simulink model "tr_trim_VTAOAS"  (R2025a)
settings: Solver=VariableStepAuto  StartTime=0.0  StopTime=10.0  RelTol=1e-3
values from neighbouring files (symbols this model uses):
  const = load_const    [vtol_trim_lin_analysis.m]
  q = X(8)    [fixedwing_6dof_dynamics.m]    (also in fixedwing_trim_dynamics.m; fw_linearization_dynamics.m; fw_trim_dynamics.m; tr_linearization_dynamics.m)
  r = X(9)    [fixedwing_6dof_dynamics.m]    (also in fixedwing_trim_dynamics.m; fw_linearization_dynamics.m; fw_trim_dynamics.m; tr_linearization_dynamics.m)
  uavParam = load_vtol_dynamics_7000lb    [vtol_trim_lin_analysis.m]
undefined symbols (not defined in the file or in its folder): contact, env, F, flap_trim, H_trim, Light, MIL, tiltIni, uavParams
libraries: matrix_library x8, robotcorelib x4, aerolibasang x2, aerolibwind2 x2, aerolibadyn x1, sharedutil x1, aerolibatmos2 x1, sharedtransform x1
(part 2 of 2)

== system tr_trim_VTAOAS/Force and Moments/Aerodynamic Forces/Compute Body Frame Forces and Moments/Wind frame F& M/Lateral Channel/Cl ==
  alpha : Inport
  beta : Inport  Port=2
  dA : Inport  Port=3
  dR : Inport  Port=4
  p,q,r : Inport  Port=5
  Airspeed : Inport  Port=6
  1-D Lookup Table : Lookup_n-D  BreakpointsForDimension1=uavParams.aero.beta_latdir  BreakpointsForDimension2=uavParams.aero.alpha_latdir  Table=uavParams.aero.CR  InternalRulePriority=Speed  RndMeth=Simplest
      settings: InputPortMap=u0,u1
  Abs : Abs  Commented=on  SaturateOnIntegerOverflow=off
  ClDa : Constant  Value=uavParams.aero.ClDa
      settings: AttributesFormatString=%<Value>
  ClDr : Constant  Value=uavParams.aero.ClDr
      settings: AttributesFormatString=%<Value>
  Clb : Constant  Commented=on  Value=uavParam.aero.Clb
      settings: AttributesFormatString=%<Value>
  Product1 : Product  SaturateOnIntegerOverflow=on  OutDataTypeStr=Inherit: Same as first input
  Product2 : Product  Commented=on
  Product5 : Product  SaturateOnIntegerOverflow=on  OutDataTypeStr=Inherit: Same as first input
  Sign : Signum  Commented=on
  Sum : Sum  Inputs=+++++  SaturateOnIntegerOverflow=on
  roll factors : Subsystem
  Cl : Outport  VectorParamsAs1DForOutWhenUnconnected=off
  wires:
  roll factors/1(Clp) -> Sum/4
  Product5/1 -> Sum/2  "CldA"
  Airspeed/1 -> roll factors/2(Airspeed)
  p,q,r/1 -> roll factors/1(p,q,r)
  roll factors/2(Clr) -> Sum/5
  Product1/1 -> Sum/3  "Cldr"
  Sum/1 -> Cl/1
  dR/1 -> Product1/2
  ClDr/1 -> Product1/1
  dA/1 -> Product5/2
  ClDa/1 -> Product5/1
  Clb/1 -> ?
  Sign/1 -> Product2/2
  1-D Lookup Table/1 -> Sum/1  "Clb"
  beta/1 -> 1-D Lookup Table/1
  alpha/1 -> 1-D Lookup Table/2

== system tr_trim_VTAOAS/Force and Moments/Aerodynamic Forces/Compute Body Frame Forces and Moments/Wind frame F& M/Lateral Channel/Cn ==
  alpha : Inport
  beta : Inport  Port=2
  dA : Inport  Port=3
  dR : Inport  Port=4
  p,q,r : Inport  Port=5
  Airspeed : Inport  Port=6
  1-D Lookup Table : Lookup_n-D  BreakpointsForDimension1=uavParams.aero.beta_latdir  BreakpointsForDimension2=uavParams.aero.alpha_latdir  Table=uavParams.aero.CN  ExtrapMethod=Clip  UseLastTableValue=on  InternalRulePriority=Speed  RndMeth=Simplest
      settings: InputPortMap=u0,u1
  Abs : Abs  Commented=on  SaturateOnIntegerOverflow=off
  CnDa : Constant  Value=uavParams.aero.CnDa
      settings: AttributesFormatString=%<Value>
  CnDr : Constant  Value=uavParams.aero.CnDr
      settings: AttributesFormatString=%<Value>
  Cnb : Constant  Commented=on  Value=uavParam.aero.Cnb
      settings: AttributesFormatString=%<Value>
  Product1 : Product  SaturateOnIntegerOverflow=on  OutDataTypeStr=Inherit: Same as first input
  Product2 : Product  Commented=on
  Product5 : Product  SaturateOnIntegerOverflow=on  OutDataTypeStr=Inherit: Same as first input
  Sign : Signum  Commented=on
  Sum : Sum  Inputs=+++++  SaturateOnIntegerOverflow=on
  yaw factors : Subsystem
  Cn : Outport  VectorParamsAs1DForOutWhenUnconnected=off
  wires:
  Airspeed/1 -> yaw factors/2(Airspeed)
  p,q,r/1 -> yaw factors/1(p,q,r)
  CnDa/1 -> Product5/1
  Product5/1 -> Sum/2
  dA/1 -> Product5/2
  CnDr/1 -> Product1/1
  dR/1 -> Product1/2
  Sum/1 -> Cn/1
  Product1/1 -> Sum/3
  yaw factors/2(Cnr) -> Sum/5
  yaw factors/1(Cnp) -> Sum/4
  1-D Lookup Table/1 -> Sum/1
  Sign/1 -> Product2/2
  alpha/1 -> 1-D Lookup Table/2
  beta/1 -> 1-D Lookup Table/1

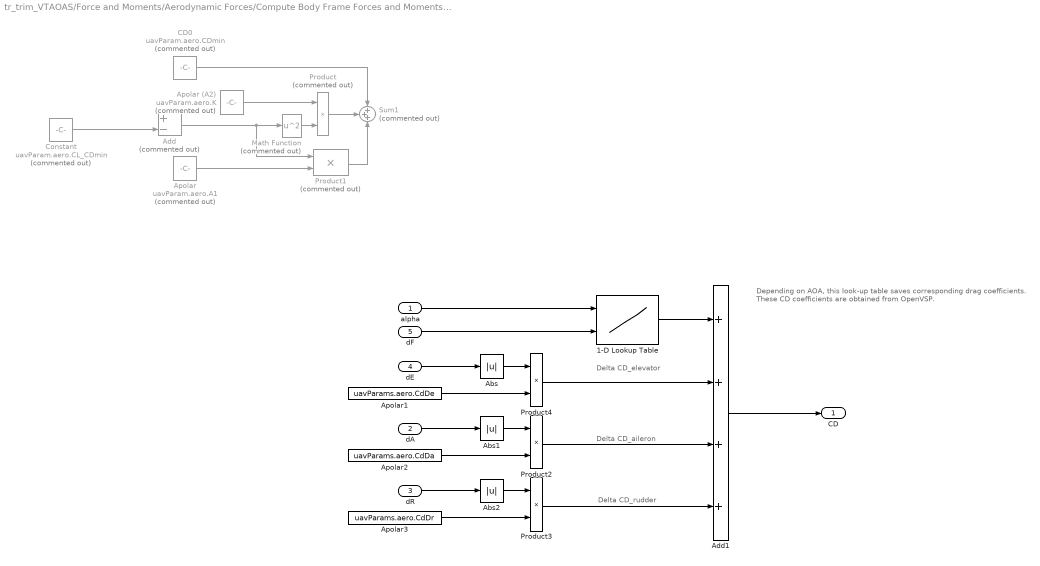
== system tr_trim_VTAOAS/Force and Moments/Aerodynamic Forces/Compute Body Frame Forces and Moments/Wind frame F& M/Longitudinal Channel/CD ==
  note: Delta CD_elevator
  note: Depending on AOA, this look-up table saves corresponding drag coefficients.
      | These CD coefficients are obtained from OpenVSP.
  note: Delta CD_aileron
  note: Delta CD_rudder
  alpha : Inport
  dA : Inport  Port=2
  dR : Inport  Port=3
  dE : Inport  Port=4
  dF : Inport  Port=5
  1-D Lookup Table : Lookup_n-D  BreakpointsForDimension1=uavParams.aero.alpha_lon  BreakpointsForDimension2=uavParams.aero.flap_lon  Table=uavParams.aero.CD  ExtrapMethod=Clip  UseLastTableValue=on  InternalRulePriority=Speed  RndMeth=Simplest
      settings: InputPortMap=u0,u1
  Abs : Abs  SaturateOnIntegerOverflow=off
  Abs1 : Abs  SaturateOnIntegerOverflow=off
  Abs2 : Abs  SaturateOnIntegerOverflow=off
  Add : Sum  Commented=on  Inputs=+-
  Add1 : Sum  Inputs=++++
  Apolar : Constant  Commented=on  Value=uavParam.aero.A1
      settings: AttributesFormatString=%<Value>
  Apolar (A2) : Constant  Commented=on  Value=uavParam.aero.K
      settings: AttributesFormatString=%<Value>
  Apolar1 : Constant  Value=uavParams.aero.CdDe
      settings: AttributesFormatString=%<Value>
  Apolar2 : Constant  Value=uavParams.aero.CdDa
      settings: AttributesFormatString=%<Value>
  Apolar3 : Constant  Value=uavParams.aero.CdDr
      settings: AttributesFormatString=%<Value>
  CD0 : Constant  Commented=on  Value=uavParam.aero.CDmin
      settings: AttributesFormatString=%<Value>
  Constant : Constant  Commented=on  Value=uavParam.aero.CL_CDmin
  Math Function : Math  Commented=on  Operator=square  SignedPower=on
  Product : Product  Commented=on  SaturateOnIntegerOverflow=on  OutDataTypeStr=Inherit: Same as first input
  Product1 : Product  Commented=on  SaturateOnIntegerOverflow=on  OutDataTypeStr=Inherit: Same as first input
  Product2 : Product  SaturateOnIntegerOverflow=on  OutDataTypeStr=Inherit: Same as first input
  Product3 : Product  SaturateOnIntegerOverflow=on  OutDataTypeStr=Inherit: Same as first input
  Product4 : Product  SaturateOnIntegerOverflow=on  OutDataTypeStr=Inherit: Same as first input
  Sum1 : Sum  Commented=on  Inputs=+++  SaturateOnIntegerOverflow=on
  CD : Outport  VectorParamsAs1DForOutWhenUnconnected=off
  wires:
  Add1/1 -> CD/1
  Apolar (A2)/1 -> Product/1
  Math Function/1 -> Product/2
  Product1/1 -> Sum1/3
  Product/1 -> Sum1/2
  Add/1 -> Product1/1, Math Function/1
  CD0/1 -> Sum1/1
  Apolar/1 -> Product1/2
  Constant/1 -> Add/2
  Apolar1/1 -> Product4/2
  dE/1 -> Abs/1
  Abs/1 -> Product4/1
  Abs1/1 -> Product2/1
  Apolar2/1 -> Product2/2
  dA/1 -> Abs1/1
  Abs2/1 -> Product3/1
  Apolar3/1 -> Product3/2
  dR/1 -> Abs2/1
  Product4/1 -> Add1/2
  Product2/1 -> Add1/3
  Product3/1 -> Add1/4
  1-D Lookup Table/1 -> Add1/1
  dF/1 -> 1-D Lookup Table/2
  alpha/1 -> 1-D Lookup Table/1

== system tr_trim_VTAOAS/Force and Moments/Aerodynamic Forces/Compute Body Frame Forces and Moments/Wind frame F& M/Longitudinal Channel/CL ==
  alpha : Inport
  alpha_dot : Inport  Port=2
  dE : Inport  Port=3
  p,q,r : Inport  Port=4
  Airspeed : Inport  Port=5
  dA : Inport  Port=6
  dF : Inport  Port=7
  1-D Lookup Table : Lookup_n-D  BreakpointsForDimension1=uavParams.aero.alpha_lon  BreakpointsForDimension2=uavParams.aero.flap_lon  Table=uavParams.aero.CL  ExtrapMethod=Clip  UseLastTableValue=on  InternalRulePriority=Speed  RndMeth=Simplest
      settings: InputPortMap=u0,u1
  Abs : Abs  SaturateOnIntegerOverflow=off
  CL1 : Constant  Value=uavParams.aero.CLDa
      settings: AttributesFormatString=%<Value>
  CLDe : Constant  Value=uavParams.aero.CLDe
      settings: AttributesFormatString=%<Value>
  CLa_dot : Constant  Value=uavParams.aero.CLadot
      settings: AttributesFormatString=%<Value>
  Lift due to pitch rate : Subsystem
  Product1 : Product  SaturateOnIntegerOverflow=on  OutDataTypeStr=Inherit: Same as first input
  Product2 : Product  SaturateOnIntegerOverflow=on  OutDataTypeStr=Inherit: Same as first input
  Product5 : Product  SaturateOnIntegerOverflow=on  OutDataTypeStr=Inherit: Same as first input
  Sum : Sum  Inputs=+++++  SaturateOnIntegerOverflow=on
  CL : Outport  VectorParamsAs1DForOutWhenUnconnected=off
  wires:
  Airspeed/1 -> Lift due to pitch rate/2(Airspeed)
  p,q,r/1 -> Lift due to pitch rate/1(p,q,r)
  Sum/1 -> CL/1
  dE/1 -> Product1/2
  CLDe/1 -> Product1/1
  alpha_dot/1 -> Product5/2
  CLa_dot/1 -> Product5/1
  CL1/1 -> Product2/2
  dA/1 -> Abs/1
  Abs/1 -> Product2/1
  Product5/1 -> Sum/2
  Lift due to pitch rate/1(CLq) -> Sum/5
  Product1/1 -> Sum/3
  Product2/1 -> Sum/4
  1-D Lookup Table/1 -> Sum/1
  alpha/1 -> 1-D Lookup Table/1
  dF/1 -> 1-D Lookup Table/2

== system tr_trim_VTAOAS/Force and Moments/Aerodynamic Forces/Compute Body Frame Forces and Moments/Wind frame F& M/Longitudinal Channel/Cm ==
  alpha : Inport
  dE : Inport  Port=2
  p,q,r : Inport  Port=3
  Airspeed : Inport  Port=4
  dF : Inport  Port=5
  1-D Lookup Table : Lookup_n-D  BreakpointsForDimension1=uavParams.aero.alpha_lon  BreakpointsForDimension2=uavParams.aero.flap_lon  Table=uavParams.aero.CM  ExtrapMethod=Clip  UseLastTableValue=on  InternalRulePriority=Speed  RndMeth=Simplest
      settings: InputPortMap=u0,u1
  CmDe : Constant  Value=uavParams.aero.CmDe
      settings: AttributesFormatString=%<Value>
  Lift due to pitch rate : Subsystem
  Product1 : Product  Inputs=**  SaturateOnIntegerOverflow=on  OutDataTypeStr=Inherit: Same as first input
  Sum : Sum  Inputs=+++  SaturateOnIntegerOverflow=on
  Cm : Outport  VectorParamsAs1DForOutWhenUnconnected=off
  wires:
  Lift due to pitch rate/1(Cmq) -> Sum/3  "cmq"
  p,q,r/1 -> Lift due to pitch rate/1(p,q,r)
  Sum/1 -> Cm/1  "total"
  dE/1 -> Product1/2
  CmDe/1 -> Product1/1
  Airspeed/1 -> Lift due to pitch rate/2(Airspeed)
  Product1/1 -> Sum/2  "cmde"
  alpha/1 -> 1-D Lookup Table/1
  1-D Lookup Table/1 -> Sum/1  "cma"
  dF/1 -> 1-D Lookup Table/2

== system tr_trim_VTAOAS/Force and Moments/Aerodynamic Forces/Compute Body Frame Forces and Moments/Wind frame F& M/Lateral Channel/CY/roll factors ==
  p,q,r : Inport
  Airspeed : Inport  Port=2
  Constant : Constant  Value=uavParams.aero.CYp
      settings: AttributesFormatString=%<Value>
  Constant1 : Constant  Value=uavParams.aero.CYr
      settings: AttributesFormatString=%<Value>
  Product : Product  SaturateOnIntegerOverflow=on  OutDataTypeStr=Inherit: Same as first input
  Product1 : Product  SaturateOnIntegerOverflow=on  OutDataTypeStr=Inherit: Same as first input
  Selector : Selector  InputPortWidth=3  IndexOptions=Index vector (dialog)  Indices=[1]  OutputSizes=1
  Selector1 : Selector  InputPortWidth=3  IndexOptions=Index vector (dialog)  Indices=[3]  OutputSizes=1
  Subsystem : Subsystem
  roll rate fact : Subsystem
  CSp : Outport  VectorParamsAs1DForOutWhenUnconnected=off
  CSr : Outport  Port=2  VectorParamsAs1DForOutWhenUnconnected=off
  wires:
  Selector1/1 -> Subsystem/1(r)
  p,q,r/1 -> Selector1/1, Selector/1
  Selector/1 -> roll rate fact/1(p)
  Airspeed/1 -> Subsystem/2(Airspeed), roll rate fact/2(Airspeed)
  Subsystem/1(Yaw Rate Fac) -> Product1/2
  roll rate fact/1(Roll Rate Fac) -> Product/2
  Product1/1 -> CSr/1
  Product/1 -> CSp/1
  Constant/1 -> Product/1
  Constant1/1 -> Product1/1

== system tr_trim_VTAOAS/Force and Moments/Aerodynamic Forces/Compute Body Frame Forces and Moments/Wind frame F& M/Lateral Channel/Cl/roll factors ==
  p,q,r : Inport
  Airspeed : Inport  Port=2
  Constant : Constant  Value=uavParams.aero.Clp
      settings: AttributesFormatString=%<Value>
  Constant1 : Constant  Value=uavParams.aero.Clr
      settings: AttributesFormatString=%<Value>
  Product : Product  SaturateOnIntegerOverflow=on  OutDataTypeStr=Inherit: Same as first input
  Product1 : Product  SaturateOnIntegerOverflow=on  OutDataTypeStr=Inherit: Same as first input
  Selector : Selector  InputPortWidth=3  IndexOptions=Index vector (dialog)  Indices=[1]  OutputSizes=1
  Selector1 : Selector  InputPortWidth=3  IndexOptions=Index vector (dialog)  Indices=[3]  OutputSizes=1
  roll rate fact : Subsystem
  yaw rate fact : Subsystem
  Clp : Outport  VectorParamsAs1DForOutWhenUnconnected=off
  Clr : Outport  Port=2  VectorParamsAs1DForOutWhenUnconnected=off
  wires:
  Selector1/1 -> yaw rate fact/1(r)
  p,q,r/1 -> Selector1/1, Selector/1
  Selector/1 -> roll rate fact/1(p)
  Airspeed/1 -> roll rate fact/2(Airspeed), yaw rate fact/2(Airspeed)
  yaw rate fact/1(Yaw Rate Fac) -> Product1/2
  Constant1/1 -> Product1/1
  roll rate fact/1(Roll Rate Fac) -> Product/2
  Constant/1 -> Product/1
  Product1/1 -> Clr/1
  Product/1 -> Clp/1

== system tr_trim_VTAOAS/Force and Moments/Aerodynamic Forces/Compute Body Frame Forces and Moments/Wind frame F& M/Lateral Channel/Cn/yaw factors ==
  p,q,r : Inport
  Airspeed : Inport  Port=2
  Constant : Constant  Value=uavParams.aero.Cnp
      settings: AttributesFormatString=%<Value>
  Constant1 : Constant  Value=uavParams.aero.Cnr
      settings: AttributesFormatString=%<Value>
  Product : Product  SaturateOnIntegerOverflow=on  OutDataTypeStr=Inherit: Same as first input
  Product1 : Product  SaturateOnIntegerOverflow=on  OutDataTypeStr=Inherit: Same as first input
  Selector : Selector  InputPortWidth=3  IndexOptions=Index vector (dialog)  Indices=[3]  OutputSizes=1
  Selector1 : Selector  InputPortWidth=3  IndexOptions=Index vector (dialog)  Indices=[1]  OutputSizes=1
  roll rate fact : Subsystem
  yaw rate fact1 : Subsystem
  Cnp : Outport  VectorParamsAs1DForOutWhenUnconnected=off
  Cnr : Outport  Port=2  VectorParamsAs1DForOutWhenUnconnected=off
  wires:
  Airspeed/1 -> yaw rate fact1/2(Airspeed), roll rate fact/2(Airspeed)
  Selector/1 -> yaw rate fact1/1(r)
  p,q,r/1 -> Selector1/1, Selector/1
  Selector1/1 -> roll rate fact/1(p)
  roll rate fact/1(Roll Rate Fac) -> Product/2
  Constant/1 -> Product/1
  yaw rate fact1/1(Yaw Rate Fac) -> Product1/2
  Constant1/1 -> Product1/1
  Product1/1 -> Cnr/1
  Product/1 -> Cnp/1

== system tr_trim_VTAOAS/Force and Moments/Aerodynamic Forces/Compute Body Frame Forces and Moments/Wind frame F& M/Longitudinal Channel/CL/Lift due to pitch rate ==
  p,q,r : Inport
  Airspeed : Inport  Port=2
  Constant : Constant  Value=uavParams.aero.CLq
      settings: AttributesFormatString=%<Value>
  Product : Product  SaturateOnIntegerOverflow=on  OutDataTypeStr=Inherit: Same as first input
  Selector : Selector  InputPortWidth=3  IndexOptions=Index vector (dialog)  Indices=[2]  OutputSizes=1
  pitch rate factor : Subsystem
  CLq : Outport  VectorParamsAs1DForOutWhenUnconnected=off
  wires:
  Airspeed/1 -> pitch rate factor/2(Airspeed)
  Selector/1 -> pitch rate factor/1(q)
  p,q,r/1 -> Selector/1
  Product/1 -> CLq/1
  pitch rate factor/1(Pitch Rate Fac) -> Product/2
  Constant/1 -> Product/1

== system tr_trim_VTAOAS/Force and Moments/Aerodynamic Forces/Compute Body Frame Forces and Moments/Wind frame F& M/Longitudinal Channel/Cm/Lift due to pitch rate ==
  p,q,r : Inport
  Airspeed : Inport  Port=2
  Constant : Constant  Value=uavParams.aero.Cmq
      settings: AttributesFormatString=%<Value>
  Product : Product  SaturateOnIntegerOverflow=on  OutDataTypeStr=Inherit: Same as first input
  Selector : Selector  InputPortWidth=3  IndexOptions=Index vector (dialog)  Indices=[2]  OutputSizes=1
  pitch rate factor : Subsystem
  Cmq : Outport  VectorParamsAs1DForOutWhenUnconnected=off
  wires:
  Airspeed/1 -> pitch rate factor/2(Airspeed)
  Selector/1 -> pitch rate factor/1(q)
  p,q,r/1 -> Selector/1
  Product/1 -> Cmq/1
  pitch rate factor/1(Pitch Rate Fac) -> Product/2
  Constant/1 -> Product/1

== system tr_trim_VTAOAS/Force and Moments/Aerodynamic Forces/Compute Body Frame Forces and Moments/Wind frame F& M/Lateral Channel/CY/roll factors/Subsystem ==
  r : Inport
  Airspeed : Inport  Port=2
  Cmq4 : Constant  Value=uavParams.geom.b
      settings: AttributesFormatString=%<Value>
  Gain : Gain  Gain=2
  Product1 : Product  Inputs=**/  SaturateOnIntegerOverflow=on  OutDataTypeStr=Inherit: Same as first input
  Saturation : Saturate  UpperLimit=inf  LowerLimit=0.1
      settings: AttributesFormatString="[%<LowerLimit>  %<UpperLimit>]"
  Yaw Rate Fac : Outport  VectorParamsAs1DForOutWhenUnconnected=off
  wires:
  Saturation/1 -> Gain/1
  Airspeed/1 -> Saturation/1
  Gain/1 -> Product1/3
  Product1/1 -> Yaw Rate Fac/1
  r/1 -> Product1/1
  Cmq4/1 -> Product1/2

== system tr_trim_VTAOAS/Force and Moments/Aerodynamic Forces/Compute Body Frame Forces and Moments/Wind frame F& M/Lateral Channel/CY/roll factors/roll rate fact ==
  p : Inport
  Airspeed : Inport  Port=2
  Cmq2 : Constant  Value=uavParams.geom.b
      settings: AttributesFormatString=%<Value>
  Gain : Gain  Gain=2
  Product : Product  Inputs=**/  SaturateOnIntegerOverflow=on  OutDataTypeStr=Inherit: Same as first input
  Saturation : Saturate  UpperLimit=inf  LowerLimit=0.1
      settings: AttributesFormatString="[%<LowerLimit>  %<UpperLimit>]"
  Roll Rate Fac : Outport  VectorParamsAs1DForOutWhenUnconnected=off
  wires:
  Airspeed/1 -> Saturation/1
  p/1 -> Product/1
  Product/1 -> Roll Rate Fac/1
  Saturation/1 -> Gain/1
  Cmq2/1 -> Product/2
  Gain/1 -> Product/3

== system tr_trim_VTAOAS/Force and Moments/Aerodynamic Forces/Compute Body Frame Forces and Moments/Wind frame F& M/Lateral Channel/Cl/roll factors/roll rate fact ==
  p : Inport
  Airspeed : Inport  Port=2
  Cmq2 : Constant  Value=uavParams.geom.b
      settings: AttributesFormatString=%<Value>
  Gain : Gain  Gain=2
  Product : Product  Inputs=**/  SaturateOnIntegerOverflow=on  OutDataTypeStr=Inherit: Same as first input
  Saturation : Saturate  UpperLimit=inf  LowerLimit=0.1
      settings: AttributesFormatString="[%<LowerLimit>  %<UpperLimit>]"
  Roll Rate Fac : Outport  VectorParamsAs1DForOutWhenUnconnected=off
  wires:
  Airspeed/1 -> Saturation/1
  p/1 -> Product/1
  Product/1 -> Roll Rate Fac/1
  Cmq2/1 -> Product/2
  Saturation/1 -> Gain/1
  Gain/1 -> Product/3

== system tr_trim_VTAOAS/Force and Moments/Aerodynamic Forces/Compute Body Frame Forces and Moments/Wind frame F& M/Lateral Channel/Cl/roll factors/yaw rate fact ==
  r : Inport
  Airspeed : Inport  Port=2
  Cmq4 : Constant  Value=uavParams.geom.b
      settings: AttributesFormatString=%<Value>
  Gain : Gain  Gain=2
  Product1 : Product  Inputs=**/  SaturateOnIntegerOverflow=on  OutDataTypeStr=Inherit: Same as first input
  Saturation : Saturate  UpperLimit=inf  LowerLimit=0.1
      settings: AttributesFormatString="[%<LowerLimit>  %<UpperLimit>]"
  Yaw Rate Fac : Outport
  wires:
  Airspeed/1 -> Saturation/1
  Saturation/1 -> Gain/1
  r/1 -> Product1/1
  Product1/1 -> Yaw Rate Fac/1
  Cmq4/1 -> Product1/2
  Gain/1 -> Product1/3

== system tr_trim_VTAOAS/Force and Moments/Aerodynamic Forces/Compute Body Frame Forces and Moments/Wind frame F& M/Lateral Channel/Cn/yaw factors/roll rate fact ==
  p : Inport
  Airspeed : Inport  Port=2
  Cmq2 : Constant  Value=uavParams.geom.b
      settings: AttributesFormatString=%<Value>
  Gain : Gain  Gain=2
  Product : Product  Inputs=**/  SaturateOnIntegerOverflow=on  OutDataTypeStr=Inherit: Same as first input
  Saturation : Saturate  UpperLimit=inf  LowerLimit=0.1
      settings: AttributesFormatString="[%<LowerLimit>  %<UpperLimit>]"
  Roll Rate Fac : Outport  VectorParamsAs1DForOutWhenUnconnected=off
  wires:
  Saturation/1 -> Gain/1
  Airspeed/1 -> Saturation/1
  p/1 -> Product/1
  Product/1 -> Roll Rate Fac/1
  Gain/1 -> Product/3
  Cmq2/1 -> Product/2

== system tr_trim_VTAOAS/Force and Moments/Aerodynamic Forces/Compute Body Frame Forces and Moments/Wind frame F& M/Lateral Channel/Cn/yaw factors/yaw rate fact1 ==
  r : Inport
  Airspeed : Inport  Port=2
  Cmq4 : Constant  Value=uavParams.geom.b
      settings: AttributesFormatString=%<Value>
  Gain : Gain  Gain=2
  Product1 : Product  Inputs=**/  SaturateOnIntegerOverflow=on  OutDataTypeStr=Inherit: Same as first input
  Saturation : Saturate  UpperLimit=inf  LowerLimit=0.1
      settings: AttributesFormatString="[%<LowerLimit>  %<UpperLimit>]"
  Yaw Rate Fac : Outport
  wires:
  Airspeed/1 -> Saturation/1
  Saturation/1 -> Gain/1
  r/1 -> Product1/1
  Product1/1 -> Yaw Rate Fac/1
  Cmq4/1 -> Product1/2
  Gain/1 -> Product1/3

== system tr_trim_VTAOAS/Force and Moments/Aerodynamic Forces/Compute Body Frame Forces and Moments/Wind frame F& M/Longitudinal Channel/CL/Lift due to pitch rate/pitch rate factor ==
  q : Inport
  Airspeed : Inport  Port=2
  Cmq2 : Constant  Value=uavParams.geom.c
      settings: AttributesFormatString=%<Value>
  Gain : Gain  Gain=2
  Product : Product  Inputs=**/  SaturateOnIntegerOverflow=on  OutDataTypeStr=Inherit: Same as first input
  Saturation : Saturate  UpperLimit=inf  LowerLimit=0.1
      settings: AttributesFormatString="[%<LowerLimit>  %<UpperLimit>]"
  Pitch Rate Fac : Outport  VectorParamsAs1DForOutWhenUnconnected=off
  wires:
  Cmq2/1 -> Product/2
  Airspeed/1 -> Saturation/1
  q/1 -> Product/1
  Product/1 -> Pitch Rate Fac/1
  Saturation/1 -> Gain/1
  Gain/1 -> Product/3

== system tr_trim_VTAOAS/Force and Moments/Aerodynamic Forces/Compute Body Frame Forces and Moments/Wind frame F& M/Longitudinal Channel/Cm/Lift due to pitch rate/pitch rate factor ==
  q : Inport
  Airspeed : Inport  Port=2
  Cmq2 : Constant  Value=uavParams.geom.c
      settings: AttributesFormatString=%<Value>
  Gain : Gain  Gain=2
  Product : Product  Inputs=**/  SaturateOnIntegerOverflow=on  OutDataTypeStr=Inherit: Same as first input
  Saturation : Saturate  UpperLimit=inf  LowerLimit=0.1
      settings: AttributesFormatString="[%<LowerLimit>  %<UpperLimit>]"
  Pitch Rate Fac : Outport  VectorParamsAs1DForOutWhenUnconnected=off
  wires:
  Cmq2/1 -> Product/2
  Airspeed/1 -> Saturation/1
  q/1 -> Product/1
  Product/1 -> Pitch Rate Fac/1
  Saturation/1 -> Gain/1
  Gain/1 -> Product/3
